simulink subsystem "Find_Target_Coordinate"  (R2023b)
settings: Solver=VariableStepAuto  StartTime=0.0  StopTime=10.0  RelTol=1e-3
undefined symbols (not defined in the file): Spline_Num_Samples
settings Model: Creator=ander  LastModifiedBy=ander

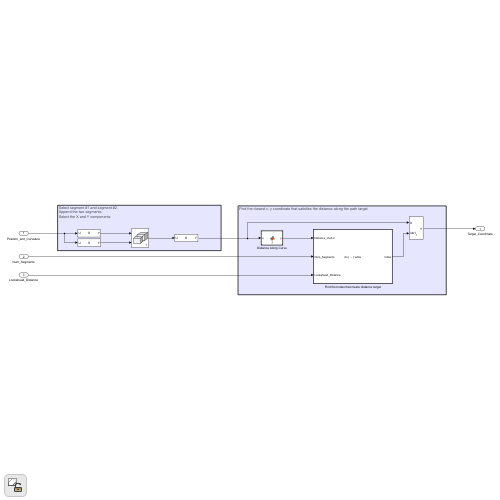
[thumbnail: Simulink's stored preview of the top-level diagram]
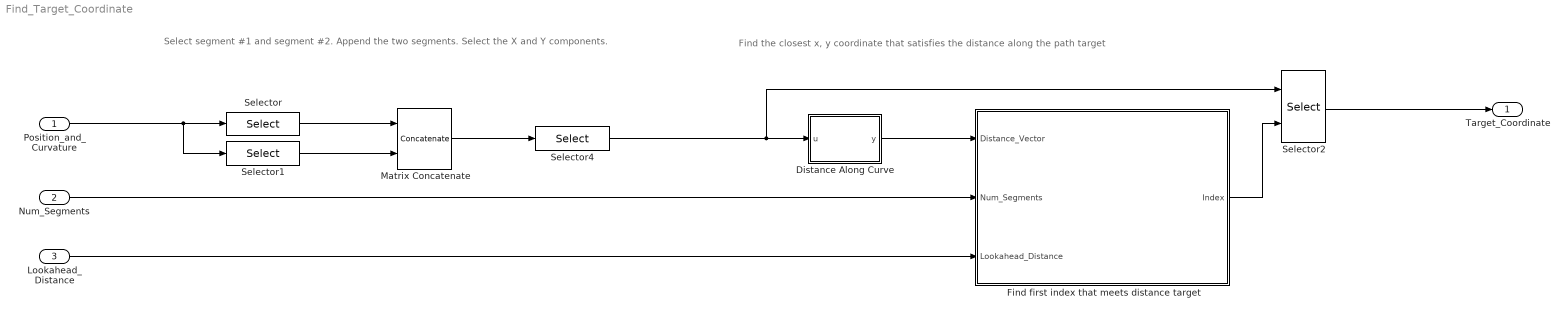
== system Find_Target_Coordinate ==
  note: Find the closest x, y coordinate that satisfies the distance along the path target
  note: Select segment #1 and segment #2.
      | Append the two segments.
      | Select the X and Y components.
  Position_and_Curvature : Inport
  Num_Segments : Inport  Port=2
  Lookahead_Distance : Inport  Port=3
  Distance Along Curve : MATLAB Function  TreatAsAtomicUnit=on
  Find first index that meets distance target : Subsystem  TreatAsAtomicUnit=on
  Matrix Concatenate : Concatenate  Mode=Multidimensional array
  Selector : Selector  NumberOfDimensions=3  InputPortWidth=3  IndexOptions=Select all,Select all,Index vector (dialog)  Indices=[1 3],1,1  OutputSizes=1,1,1
  Selector1 : Selector  NumberOfDimensions=3  InputPortWidth=3  IndexOptions=Select all,Select all,Index vector (dialog)  Indices=[1 3],1,2  OutputSizes=1,1,1
  Selector2 : Selector  NumberOfDimensions=2  InputPortWidth=Spline_Num_Samples_x2  IndexOptions=Index vector (port),Select all  Indices=[1 3],1  OutputSizes=1,1
  Selector4 : Selector  NumberOfDimensions=2  InputPortWidth=3  IndexOptions=Select all,Index vector (dialog)  Indices=[1 3],[1 2]  OutputSizes=1,1
  Target_Coordinate : Outport
  wires:
  Position_and_Curvature/1 -> Selector/1, Selector1/1
  Selector1/1 -> Matrix Concatenate/2
  Matrix Concatenate/1 -> Selector4/1
  Selector/1 -> Matrix Concatenate/1
  Selector2/1 -> Target_Coordinate/1
  Selector4/1 -> Selector2/1, Distance Along Curve/1(u)
  Distance Along Curve/1(y) -> Find first index that meets distance target/1(Distance_Vector)
  Find first index that meets distance target/1(Index) -> Selector2/2
  Lookahead_Distance/1 -> Find first index that meets distance target/3(Lookahead_Distance)
  Num_Segments/1 -> Find first index that meets distance target/2(Num_Segments)

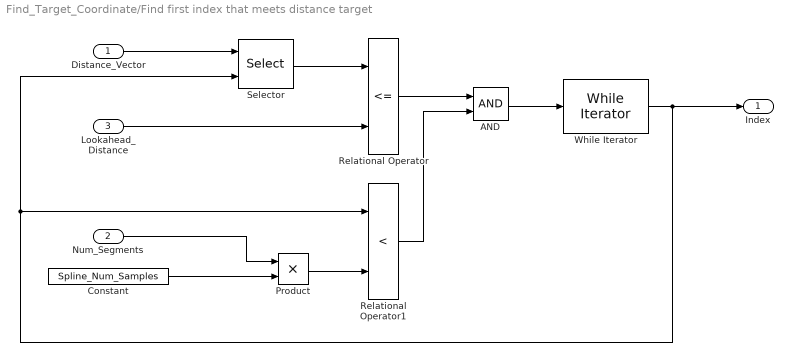
== system Find_Target_Coordinate/Find first index that meets distance target ==
  Distance_Vector : Inport
  Num_Segments : Inport  Port=2
  Lookahead_Distance : Inport  Port=3
  AND : Logic  AllPortsSameDT=off  OutDataTypeStr=boolean
  Constant : Constant  Value=Spline_Num_Samples
  Product : Product
  Relational Operator : RelationalOperator  Operator=<=  OutDataTypeStr=boolean  RndMeth=Simplest  InputSameDT=off
  Relational Operator1 : RelationalOperator  Operator=<  OutDataTypeStr=boolean  RndMeth=Simplest  InputSameDT=off
  Selector : Selector  InputPortWidth=Spline_Num_Samples_x2  IndexOptions=Index vector (port)  Indices=[1 3]  OutputSizes=1
  While Iterator : WhileIterator  MaxIters=Spline_Num_Samples_x2  WhileBlockType=do-while  ResetStates=reset  ShowIterationPort=on  OutputDataType=uint8
  Index : Outport
  wires:
  AND/1 -> While Iterator/1
  Relational Operator/1 -> AND/1
  Relational Operator1/1 -> AND/2
  Constant/1 -> Product/2
  Num_Segments/1 -> Product/1
  Product/1 -> Relational Operator1/2
  While Iterator/1 -> Index/1, Relational Operator1/1, Selector/2
  Lookahead_Distance/1 -> Relational Operator/2
  Selector/1 -> Relational Operator/1
  Distance_Vector/1 -> Selector/1

== matlab function Find_Target_Coordinate/Distance Along Curve ==
  data: u input; y output
function y = distance(u)
% u = input matrix of dimension [length x 2]
%     where the first column is the x coordinate
%     where the second column is the y coordinate
% y = distance along the x, y coordinate path
%     assuming straight line distances between points

len = length(u);
distance_sum = zeros(len,1);
for k = 2:len
    x_delta = u(k,1)-u(k-1,1);
    y_delta = u(k,2)-u(k-1,2);
    distance = hypot(x_delta,y_delta);
    distance_sum(k) = distance_sum(k-1) + distance;
end

y = distance_sum;
